simulink model "Caso8PInaolinear"  (R2015a)
settings: Solver=ode45  StartTime=0.0  StopTime=60  RelTol=1e-3
settings Model: Creator=user  LastModifiedBy=user

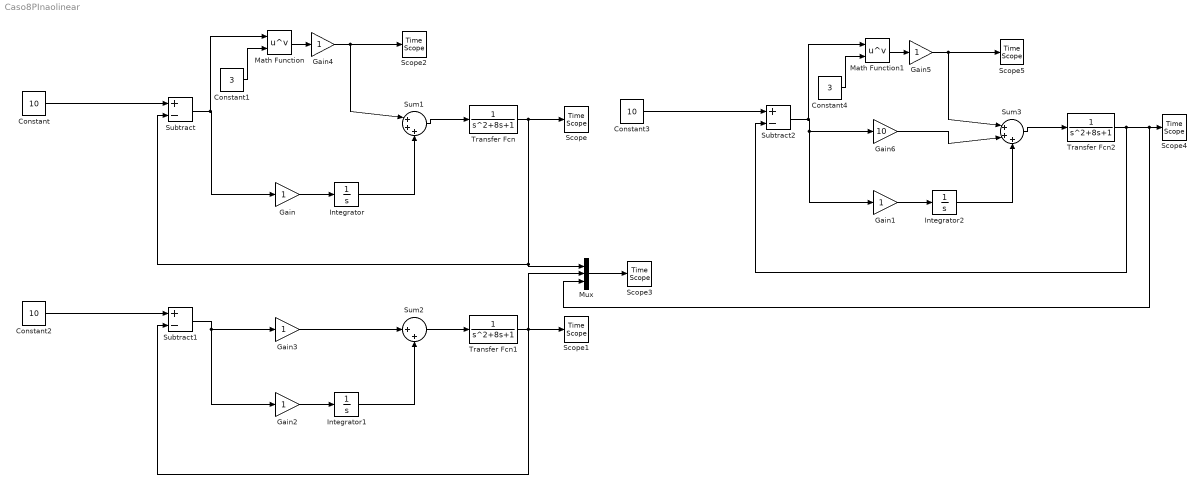
== system Caso8PInaolinear ==
  Constant : Constant  Value=10
  Constant1 : Constant  Value=3
  Constant2 : Constant  Value=10
  Constant3 : Constant  Value=10
  Constant4 : Constant  Value=3
  Gain{,1..5} (6 alike) : Gain
  Gain6 : Gain  Gain=10
  Integrator : Integrator
  Integrator1 : Integrator
  Integrator2 : Integrator
  Math Function : Math  Operator=pow  SaturateOnIntegerOverflow=on
  Math Function1 : Math  Operator=pow  SaturateOnIntegerOverflow=on
  Mux : Mux  Inputs=3
  Scope{,1..5} (6 alike) : TimeScope
  Subtract : Sum  Inputs=+-
  Subtract1 : Sum  Inputs=+-
  Subtract2 : Sum  Inputs=+-
  Sum1 : Sum  Inputs=|+++
  Sum2 : Sum  Inputs=|++
  Sum3 : Sum  Inputs=|+++
  Transfer Fcn : TransferFcn  Denominator=[1 8 1]
  Transfer Fcn1 : TransferFcn  Denominator=[1 8 1]
  Transfer Fcn2 : TransferFcn  Denominator=[1 8 1]
  wires:
  Gain/1 -> Integrator/1
  Transfer Fcn/1 -> Scope/1, Mux/1, Subtract/2
  Sum1/1 -> Transfer Fcn/1
  Constant/1 -> Subtract/1
  Subtract/1 -> Math Function/1, Gain/1
  Integrator/1 -> Sum1/3
  Math Function/1 -> Gain4/1
  Gain2/1 -> Integrator1/1
  Transfer Fcn1/1 -> Mux/2, Scope1/1, Subtract1/2
  Sum2/1 -> Transfer Fcn1/1
  Constant2/1 -> Subtract1/1
  Subtract1/1 -> Gain2/1, Gain3/1
  Integrator1/1 -> Sum2/2
  Gain3/1 -> Sum2/1
  Gain4/1 -> Sum1/1, Scope2/1
  Constant1/1 -> Math Function/2
  Mux/1 -> Scope3/1
  Gain1/1 -> Integrator2/1
  Transfer Fcn2/1 -> Mux/3, Scope4/1, Subtract2/2
  Sum3/1 -> Transfer Fcn2/1
  Constant3/1 -> Subtract2/1
  Subtract2/1 -> Math Function1/1, Gain6/1, Gain1/1
  Integrator2/1 -> Sum3/3
  Math Function1/1 -> Gain5/1
  Gain5/1 -> Sum3/1, Scope5/1
  Constant4/1 -> Math Function1/2
  Gain6/1 -> Sum3/2
